simulink model "creazioneVettorea"  (R2021a)
settings: Solver=VariableStepAuto  StartTime=0.0  StopTime=1
settings Model: Creator=Benedetta  LastModifiedBy=Benedetta

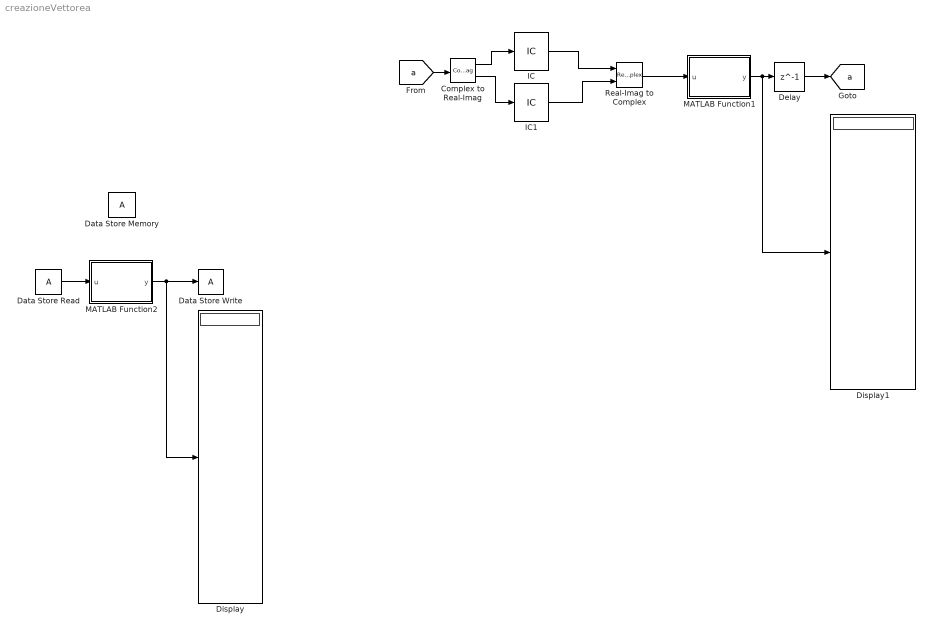
== system creazioneVettorea ==
  Complex to Real-Imag : ComplexToRealImag
  Data Store Memory : DataStoreMemory  ReadBeforeWriteMsg=warning  WriteAfterWriteMsg=warning  WriteAfterReadMsg=warning  InitialValue=ones(1,20) + 1i*zeros(1,20)  ShowAdditionalParam=off
      settings: SignalType=complex
  Data Store Read : DataStoreRead  SampleTime=0.01  IndexOptions=Index vector (dialog)  Indices=1  OutputSizes=1
  Data Store Write : DataStoreWrite  SampleTime=0.01  IndexOptions=Index vector (dialog)  Indices=1  OutputSizes=1
  Delay : Delay  DelayLength=1
  Display : Display
  Display1 : Display
  IC : InitialCondition  Value=ones(1,20)
  IC1 : InitialCondition  Value=zeros(1,20)
  MATLAB Function1 : MATLAB Function  TreatAsAtomicUnit=on
  MATLAB Function2 : MATLAB Function  TreatAsAtomicUnit=on
  Real-Imag to Complex : RealImagToComplex
  tag scope: a=global
  wires:
  [a] -> Complex to Real-Imag/1
  Complex to Real-Imag/1 -> IC/1
  Complex to Real-Imag/2 -> IC1/1
  IC/1 -> Real-Imag to Complex/1
  IC1/1 -> Real-Imag to Complex/2
  Real-Imag to Complex/1 -> MATLAB Function1/1(u)
  MATLAB Function1/1(y) -> Display1/1, Delay/1
  Delay/1 -> [a]
  Data Store Read/1 -> MATLAB Function2/1(u)
  MATLAB Function2/1(y) -> Display/1, Data Store Write/1

== matlab function creazioneVettorea/MATLAB Function2 ==
  data: u input; y output
function y = fcn(u)
i = 5; 
u_new = u;
u_new(i) = 10; 
y = u_new;

== matlab function creazioneVettorea/MATLAB Function1 ==
  data: u input; y output
function y = fcn(u)
i = 5; 
u_new = u;
u_new(i) = 10; 
y = u_new
